simulink model "data_acquisition"  (R2023b)
settings: Solver=FixedStepDiscrete  StartTime=0.0  StopTime=Inf  RelTol=1e-3  EnableMultiTasking=on
libraries: c2802xlib x4
settings Model: SimulationMode=external  ExtModeTrigDuration=8  Creator=Yamukelani  LastModifiedBy=yamzi
settings SolverCC: AutoInsertRateTranBlk=on
settings DataIOCC: LoggingToFile=on  LoggingFileName=C:\Users\yamzi\source_code\msc_research\rul_prediction\src\datasets\msc_rul_data.mat
settings OptimizationCC: UseDivisionForNetSlopeComputation=on  GainParamInheritBuiltInType=on  UseFloatMulNetSlope=on  DefaultUnderspecifiedDataType=single  EnhancedBackFolding=on  PassReuseOutputArgsAs=Individual arguments  EfficientFloat2IntCast=on  MaxStackSize=768  OptimizeBlockOrder=speed  DifferentSizesBufferReuse=on  OptimizationCustomize=off  EfficientTunableParamExpr=on
settings DebuggingCC: ParameterTunabilityLossMsg=error  UniqueDataStoreMsg=error
settings HardwareCC: ProdBitPerChar=16  ProdBitPerInt=16  ProdBitPerPointer=32  ProdBitPerSizeT=32  ProdBitPerPtrDiffT=32  ProdLargestAtomicInteger=Integer  ProdLargestAtomicFloat=None  ProdWordSize=16  ProdLongLongMode=on  ProdHWDeviceType=Texas Instruments->C2000  TargetBitPerPointer=64  TargetBitPerSizeT=64  TargetBitPerPtrDiffT=64  TargetLongLongMode=on  TargetIntDivRoundTo=Zero  TargetEndianess=LittleEndian  TargetWordSize=64  TargetHWDeviceType=MATLAB Host  ProdEqTarget=off
settings ModelReferenceCC: ModelReferenceNumInstancesAllowed=Single
settings SFSimCC: SimCustomHeaderCode="#include \"F2802x_Device.h\""  SimParseCustomCode=off  MATLABDynamicMemAlloc=off
settings SFSimCC: SimUserIncludeDirs=|
  | C:\ti\c2000\C2000Ware_5_01_00_00\device_support\f2802x\headers\include
  | C:\ti\c2000\C2000Ware_5_01_00_00\device_support\f2802x\common\source
settings RTWCC: Description=Embedded Coder  SystemTargetFile=ert.tlc  HardwareBoard=TI Piccolo F2802x  TemplateMakefile=ert_default_tmf  GenerateReport=on  CustomHeaderCode="#include \"F2802x_Device.h\""  Toolchain=Texas Instruments Code Composer Studio (C2000)  LaunchReport=on  CodeProfilingSaveOptions=MetricsOnly
settings RTWCC: CustomInclude=|
  | C:\ti\c2000\C2000Ware_5_01_00_00\device_support\f2802x\headers\include
  | C:\ti\c2000\C2000Ware_5_01_00_00\device_support\f2802x\common\source
settings RTWCC: CustomSource=|
  | "C:\ti\c2000\C2000Ware_5_01_00_00\device_support\f2802x\common\source\pll.c"
  | "C:\ti\c2000\C2000Ware_5_01_00_00\device_support\f2802x\common\source\pwm.c"
  | "C:\ti\c2000\C2000Ware_5_01_00_00\device_support\f2802x\common\source\pwr.c"
  | "C:\ti\c2000\C2000Ware_5_01_00_00\device_support\f2802x\common\source\sci.c"
  | "C:\ti\c2000\C2000Ware_5_01_00_00\device_support\f2802x\common\source\sci_io.c"
  | "C:\ti\c2000\C2000Ware_5_01_00_00\device_support\f2802x\common\source\spi.c"
  | "C:\ti\c2000\C2000Ware_5_01_00_00\device_support\f2802x\common\source\timer.c"
  | "C:\ti\c2000\C2000Ware_5_01_00_00\device_support\f2802x\common\source\wdog.c"
  | "C:\ti\c2000\C2000Ware_5_01_00_00\device_support\f2802x\common\source\gpio.c"
  | "C:\ti\c2000\C2000Ware_5_01_00_00\device_support\f2802x\common\source\i2c.c"
  | "C:\ti\c2000\C2000Ware_5_01_00_00\device_support\f2802x\common\source\osc.c"
  | "C:\ti\c2000\C2000Ware_5_01_00_00\device_support\f2802x\common\source\pie.c"
  | "C:\ti\c2000\C2000Ware_5_01_00_00\device_support\f2802x\common\source\f2802x_pievect.c"
  | "C:\ti\c2000\C2000Ware_5_01_00_00\device_support\f2802x\common\source\f2802x_sci.c"
  | "C:\ti\c2000\C2000Ware_5_01_00_00\device_support\f2802x\common\source\f2802x_spi.c"
  | "C:\ti\c2000\C2000Ware_5_01_00_00\device_support\f2802x\common\source\f2802x_ecap.c"
  | "C:\ti\c2000\C2000Ware_5_01_00_00\device_support\f2802x\common\source\f2802x_epwm.c"
  | "C:\ti\c2000\C2000Ware_5_01_00_00\device_support\f2802x\common\source\f2802x_gpio.c"
  | "C:\ti\c2000\C2000Ware_5_01_00_00\device_support\f2802x\common\source\f2802x_i2c.c"
  | "C:\ti\c2000\C2000Ware_5_01_00_00\device_support\f2802x\common\source\f2802x_osccomp.c"
  | "C:\ti\c2000\C2000Ware_5_01_00_00\device_support\f2802x\common\source\f2802x_piectrl.c"
settings RTWCC: CustomInitializer=|
  | #ifndef MATLAB_MEX_FILE
  | #include "F2802x_Device.h"
  | #endif
settings CodeAppCC: ForceParamTrailComments=on  IgnoreCustomStorageClasses=off  OperatorAnnotations=on  SimulinkDataObjDesc=on  SFDataObjDesc=on  InsertBlockDesc=on
settings ERTTargetCC: TargetLangStandard=C99 (ISO)  ExtModeTransport=4  ExtModeStaticAlloc=on  ExtModeAutomaticAllocSize=off  ExtModeStaticAllocSize=500  ExtModeMexFile=ext_xcp  ExtModeIntrfLevel=Level2 - Open
settings ConfigComp: CovScope=ReferencedModels

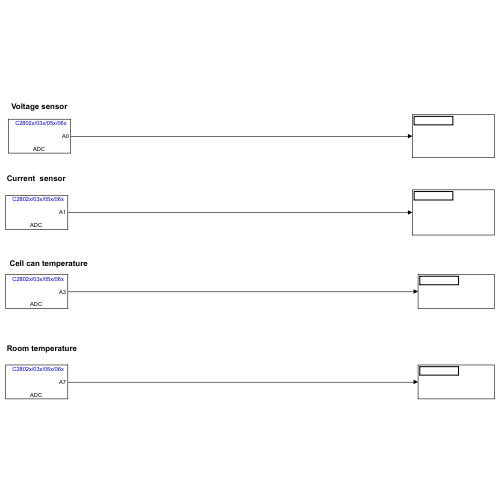
[thumbnail: Simulink's stored preview of the top-level diagram]
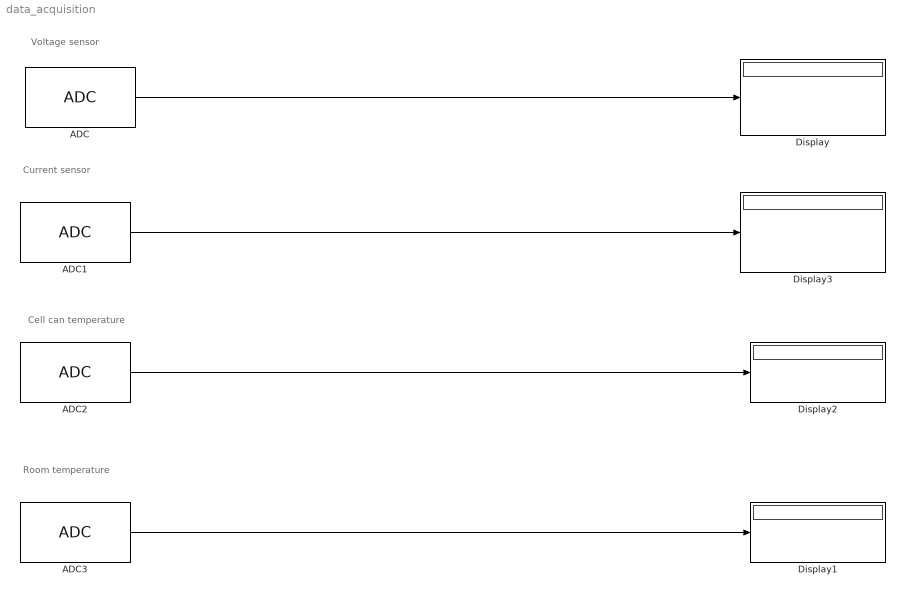
== system data_acquisition ==
  note: Current sensor
  note: Voltage sensor
  note: Cell can temperature
  note: Room temperature
  ADC : c2802xlib/ADC  blkParamProc=C2000  ADCModule=1  samplingMode=Single sample mode  ADCResolution=12-bit (Single-ended input)  useSOC1=SOC0  useSOC2=SOC0_SOC1  SOCAcquisitionWindow=7  SOCTriggerSource=CPU0_TINT0n  SOCInterruptTrigger=No ADCINT  Ts=0.005  dType=uint16  postInterrupt=off  interruptSel=ADCINT1  ADCINTContinuous=on  endma=off  chdma=1  conv1=ADCINA0  conv2=ADCINA0 and ADCINB0  conv1_Type4=ADCIN0  conv2_Type4=ADCIN0 and ADCIN1
  ADC1 : c2802xlib/ADC  blkParamProc=C2000  ADCModule=1  samplingMode=Single sample mode  ADCResolution=12-bit (Single-ended input)  useSOC1=SOC1  useSOC2=SOC0_SOC1  SOCAcquisitionWindow=7  SOCTriggerSource=CPU0_TINT0n  SOCInterruptTrigger=No ADCINT  Ts=0.005  dType=uint16  postInterrupt=off  interruptSel=ADCINT1  ADCINTContinuous=on  endma=off  chdma=1  conv1=ADCINA1  conv2=ADCINA0 and ADCINB0  conv1_Type4=ADCIN0  conv2_Type4=ADCIN0 and ADCIN1
  ADC2 : c2802xlib/ADC  blkParamProc=C2000  ADCModule=1  samplingMode=Single sample mode  ADCResolution=12-bit (Single-ended input)  useSOC1=SOC2  useSOC2=SOC0_SOC1  SOCAcquisitionWindow=7  SOCTriggerSource=CPU0_TINT0n  SOCInterruptTrigger=No ADCINT  Ts=0.005  dType=uint16  postInterrupt=off  interruptSel=ADCINT1  ADCINTContinuous=on  endma=off  chdma=1  conv1=ADCINA3  conv2=ADCINA0 and ADCINB0  conv1_Type4=ADCIN0  conv2_Type4=ADCIN0 and ADCIN1
  ADC3 : c2802xlib/ADC  blkParamProc=C2000  ADCModule=1  samplingMode=Single sample mode  ADCResolution=12-bit (Single-ended input)  useSOC1=SOC3  useSOC2=SOC0_SOC1  SOCAcquisitionWindow=7  SOCTriggerSource=CPU0_TINT0n  SOCInterruptTrigger=No ADCINT  Ts=0.005  dType=uint16  postInterrupt=off  interruptSel=ADCINT1  ADCINTContinuous=on  endma=off  chdma=1  conv1=ADCINA7  conv2=ADCINA0 and ADCINB0  conv1_Type4=ADCIN0  conv2_Type4=ADCIN0 and ADCIN1
  Display{,1..3} (4 alike) : Display
  wires:
  ADC/1 -> Display/1
  ADC1/1 -> Display3/1
  ADC2/1 -> Display2/1
  ADC3/1 -> Display1/1
